simulink model "Simulink_VDP"  (R2022a)
settings: Solver=FixedStepAuto  StartTime=0.0  StopTime=10.0  FixedStep=ts  RelTol=1e-3
libraries: mpclib x1
settings Model: Creator=sergiovaneg  LastModifiedBy=sergiovaneg

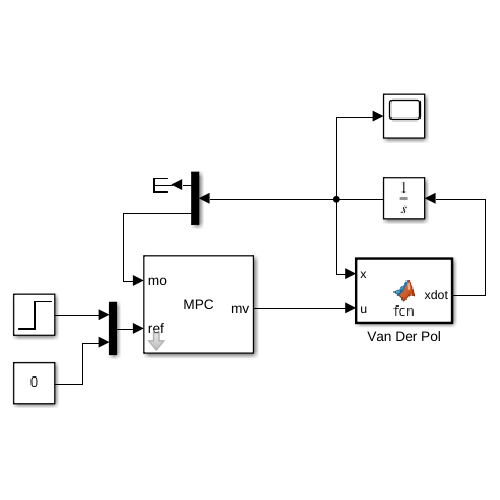
[thumbnail: Simulink's stored preview of the top-level diagram]
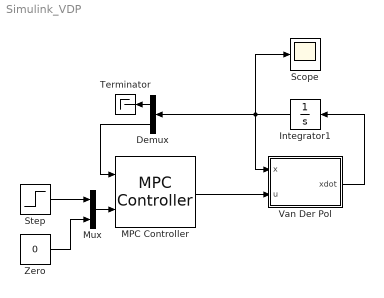
== system Simulink_VDP ==
  Demux : Demux  Outputs=2
  Integrator1 : Integrator
  MPC Controller : mpclib/MPC Controller  SCDEnableBlockLinearizationSpecification=on  is_multiple=0  enable_value=0  return_u0=off  updateMPCinCallerWorkspace=on  md_inport=off  mv_inport=off  uref_inport=off  return_cost=off  return_mvseq=off  return_qpstatus=off  return_xseq=off  return_state=off  return_ovseq=off  state_inport=off  umin_inport=off  umax_inport=off  ymin_inport=off  ymax_inport=off  cc_inport=off  ywt_inport=off  uwt_inport=off  duwt_inport=off  rhoeps_inport=off  pm_inport=off  MaximumP=10  HorizonChoice=FixedHorizon  n_ts=1  n_p=10  n_mv=1  n_md=1  n_ud=0  n_mo=1  n_uo=0  BlockDataType=double  SampleTimeInherited=off  switch_inport=off
  Mux : Mux  Inputs=2
  Scope : Scope
  Step : Step  SampleTime=0
  Terminator : Terminator
  Van Der Pol : MATLAB Function  TreatAsAtomicUnit=on
  Zero : Constant  Value=0  OutDataTypeStr=Inherit: Inherit via back propagation
  wires:
  Van Der Pol/1(xdot) -> Integrator1/1
  Integrator1/1 -> Scope/1, Demux/1, Van Der Pol/1(x)
  MPC Controller/1 -> Van Der Pol/2(u)
  Demux/2 -> MPC Controller/1
  Demux/1 -> Terminator/1
  Mux/1 -> MPC Controller/2
  Step/1 -> Mux/1
  Zero/1 -> Mux/2

== matlab function Simulink_VDP/Van Der Pol ==
  data: x input; u input; xdot output
function xdot = fcn(x,u)

xdot = [2*x(2);
        -0.8*x(1)+2*x(2)-10*(x(1)^2)*x(2) + u];
